simulink subsystem "AeroPropRefFranc"  (R2024b)
settings: Solver=VariableStepAuto  StartTime=0.0  StopTime=10.0  RelTol=1e-3
undefined symbols (not defined in the file or in its folder): ess, Force_b, Fprop_r, geom, H_b, Hdot_b, Moment_b, mot, mot2, mot3, mot4, Mprop_r, propel, propel2, propel3, propel4, pxf_diagram_options, SimIn, SimPar, tc, tc2, tc3, tc4
libraries: simulink x8, slpidlib x4, starslibAxisTransformations x2, libAxisTransformations x2
(part 2 of 10)

== system AeroPropRefFranc/Propulsion and Aerodynamic Forces and Moments/S-Function/Battery Model/powerplant/mot2 ==
  main_info_bus_in : Inport
  system_effort_in : Inport  Port=2
  system_flow_in : Inport  Port=3
  buscreator_system_bus_out1 : BusCreator  Inputs=2
  ctrl : Subsystem
  memoryctrl : Memory
  plant : Subsystem
      mask Display: disp('mot2_plant_map_Pelec_funTW_volt_in.slx')
  system_bus_out : Outport
  system_effort_out : Outport  Port=2
  system_flow_out : Outport  Port=3
  wires:
  [plant] -> buscreator_system_bus_out1/2  "plant"
  [ctrl] -> buscreator_system_bus_out1/1  "ctrl"
  buscreator_system_bus_out1/1 -> system_bus_out/1  "system_info_bus"
  system_flow_in/1 -> plant/4(in-flow-3)  "flow"
  system_effort_in/1 -> plant/3(in-effort-2)  "effort"
  plant/4(out-flow-8) -> system_flow_out/1  "flow"
  plant/3(out-effort-7) -> system_effort_out/1  "effort"
  plant/1(outport-system_info_bus) -> [plant]  "system_info_bus"
  memoryctrl/1 -> plant/2(inport-ctrl_bus-2)  "ctrl_bus"
  plant/2(outport-plant_bus) -> ctrl/2(local_info_bus_in)  "plant_bus"
  main_info_bus_in/1 -> plant/1(aInport--1), ctrl/1(main_info_bus_in)  "main_info_bus"
  ctrl/2(local_info_bus_out) -> memoryctrl/1  "ctrl_bus"
  ctrl/1(system_bus_out) -> [ctrl]  "system_info_bus"

== system AeroPropRefFranc/Propulsion and Aerodynamic Forces and Moments/S-Function/Battery Model/powerplant/mot3 ==
  main_info_bus_in : Inport
  system_effort_in : Inport  Port=2
  system_flow_in : Inport  Port=3
  buscreator_system_bus_out1 : BusCreator  Inputs=2
  ctrl : Subsystem
  memoryctrl : Memory
  plant : Subsystem
      mask Display: disp('mot3_plant_map_Pelec_funTW_volt_in.slx')
  system_bus_out : Outport
  system_effort_out : Outport  Port=2
  system_flow_out : Outport  Port=3
  wires:
  [plant] -> buscreator_system_bus_out1/2  "plant"
  [ctrl] -> buscreator_system_bus_out1/1  "ctrl"
  buscreator_system_bus_out1/1 -> system_bus_out/1  "system_info_bus"
  system_flow_in/1 -> plant/4(in-flow-3)  "flow"
  system_effort_in/1 -> plant/3(in-effort-2)  "effort"
  plant/4(out-flow-8) -> system_flow_out/1  "flow"
  plant/3(out-effort-7) -> system_effort_out/1  "effort"
  plant/1(outport-system_info_bus) -> [plant]  "system_info_bus"
  memoryctrl/1 -> plant/2(inport-ctrl_bus-2)  "ctrl_bus"
  plant/2(outport-plant_bus) -> ctrl/2(local_info_bus_in)  "plant_bus"
  main_info_bus_in/1 -> plant/1(aInport--1), ctrl/1(main_info_bus_in)  "main_info_bus"
  ctrl/2(local_info_bus_out) -> memoryctrl/1  "ctrl_bus"
  ctrl/1(system_bus_out) -> [ctrl]  "system_info_bus"

== system AeroPropRefFranc/Propulsion and Aerodynamic Forces and Moments/S-Function/Battery Model/powerplant/mot4 ==
  main_info_bus_in : Inport
  system_effort_in : Inport  Port=2
  system_flow_in : Inport  Port=3
  buscreator_system_bus_out1 : BusCreator  Inputs=2
  ctrl : Subsystem
  memoryctrl : Memory
  plant : Subsystem
      mask Display: disp('mot4_plant_map_Pelec_funTW_volt_in.slx')
  system_bus_out : Outport
  system_effort_out : Outport  Port=2
  system_flow_out : Outport  Port=3
  wires:
  [plant] -> buscreator_system_bus_out1/2  "plant"
  [ctrl] -> buscreator_system_bus_out1/1  "ctrl"
  buscreator_system_bus_out1/1 -> system_bus_out/1  "system_info_bus"
  system_flow_in/1 -> plant/4(in-flow-3)  "flow"
  system_effort_in/1 -> plant/3(in-effort-2)  "effort"
  plant/4(out-flow-8) -> system_flow_out/1  "flow"
  plant/3(out-effort-7) -> system_effort_out/1  "effort"
  plant/1(outport-system_info_bus) -> [plant]  "system_info_bus"
  memoryctrl/1 -> plant/2(inport-ctrl_bus-2)  "ctrl_bus"
  plant/2(outport-plant_bus) -> ctrl/2(local_info_bus_in)  "plant_bus"
  main_info_bus_in/1 -> plant/1(aInport--1), ctrl/1(main_info_bus_in)  "main_info_bus"
  ctrl/2(local_info_bus_out) -> memoryctrl/1  "ctrl_bus"
  ctrl/1(system_bus_out) -> [ctrl]  "system_info_bus"

== system AeroPropRefFranc/Propulsion and Aerodynamic Forces and Moments/S-Function/Battery Model/powerplant/propel ==
  main_info_bus_in : Inport
  system_effort_in : Inport  Port=2
  system_flow_in : Inport  Port=3
  Ground_1 : Ground
  Terminator_1 : Terminator
  plant : Subsystem
      mask Display: disp('propel_plant_uas.slx')
  system_bus_out : Outport
  system_effort_out : Outport  Port=2
  system_flow_out : Outport  Port=3
  wires:
  plant/2(aOutport--2) -> Terminator_1/1
  Ground_1/1 -> plant/2(aInport--2)
  [plant] -> system_bus_out/1  "plant"
  system_flow_in/1 -> plant/4(in-flow-5)
  system_effort_in/1 -> plant/3(in-effort-4)
  plant/4(out-flow-6) -> system_flow_out/1
  plant/3(out-effort-5) -> system_effort_out/1
  plant/1(outport-system_info_bus) -> [plant]
  main_info_bus_in/1 -> plant/1(inport-main_info_bus-1)

== system AeroPropRefFranc/Propulsion and Aerodynamic Forces and Moments/S-Function/Battery Model/powerplant/propel2 ==
  main_info_bus_in : Inport
  system_effort_in : Inport  Port=2
  system_flow_in : Inport  Port=3
  Ground_1 : Ground
  Terminator_1 : Terminator
  plant : Subsystem
      mask Display: disp('propel2_plant_uas.slx')
  system_bus_out : Outport
  system_effort_out : Outport  Port=2
  system_flow_out : Outport  Port=3
  wires:
  plant/2(aOutport--2) -> Terminator_1/1
  Ground_1/1 -> plant/2(aInport--2)
  [plant] -> system_bus_out/1  "plant"
  system_flow_in/1 -> plant/4(in-flow-5)
  system_effort_in/1 -> plant/3(in-effort-4)
  plant/4(out-flow-6) -> system_flow_out/1
  plant/3(out-effort-5) -> system_effort_out/1
  plant/1(outport-system_info_bus) -> [plant]
  main_info_bus_in/1 -> plant/1(inport-main_info_bus-1)

== system AeroPropRefFranc/Propulsion and Aerodynamic Forces and Moments/S-Function/Battery Model/powerplant/propel3 ==
  main_info_bus_in : Inport
  system_effort_in : Inport  Port=2
  system_flow_in : Inport  Port=3
  Ground_1 : Ground
  Terminator_1 : Terminator
  plant : Subsystem
      mask Display: disp('propel3_plant_uas.slx')
  system_bus_out : Outport
  system_effort_out : Outport  Port=2
  system_flow_out : Outport  Port=3
  wires:
  plant/2(aOutport--2) -> Terminator_1/1
  Ground_1/1 -> plant/2(aInport--2)
  [plant] -> system_bus_out/1  "plant"
  system_flow_in/1 -> plant/4(in-flow-5)
  system_effort_in/1 -> plant/3(in-effort-4)
  plant/4(out-flow-6) -> system_flow_out/1
  plant/3(out-effort-5) -> system_effort_out/1
  plant/1(outport-system_info_bus) -> [plant]
  main_info_bus_in/1 -> plant/1(inport-main_info_bus-1)

== system AeroPropRefFranc/Propulsion and Aerodynamic Forces and Moments/S-Function/Battery Model/powerplant/propel4 ==
  main_info_bus_in : Inport
  system_effort_in : Inport  Port=2
  system_flow_in : Inport  Port=3
  Ground_1 : Ground
  Terminator_1 : Terminator
  plant : Subsystem
      mask Display: disp('propel4_plant_uas.slx')
  system_bus_out : Outport
  system_effort_out : Outport  Port=2
  system_flow_out : Outport  Port=3
  wires:
  plant/2(aOutport--2) -> Terminator_1/1
  Ground_1/1 -> plant/2(aInport--2)
  [plant] -> system_bus_out/1  "plant"
  system_flow_in/1 -> plant/4(in-flow-5)
  system_effort_in/1 -> plant/3(in-effort-4)
  plant/4(out-flow-6) -> system_flow_out/1
  plant/3(out-effort-5) -> system_effort_out/1
  plant/1(outport-system_info_bus) -> [plant]
  main_info_bus_in/1 -> plant/1(inport-main_info_bus-1)

== system AeroPropRefFranc/Propulsion and Aerodynamic Forces and Moments/S-Function/Battery Model/powerplant/tc ==
  main_info_bus_in : Inport
  system_effort_in : Inport  Port=2
  system_flow_in : Inport  Port=3
  Ground_1 : Ground
  Terminator_1 : Terminator
  plant : Subsystem
      mask Display: disp('tc_plant_map_trqloss_funTW.slx')
  system_bus_out : Outport
  system_effort_out : Outport  Port=2
  system_flow_out : Outport  Port=3
  wires:
  plant/2(aOutport--2) -> Terminator_1/1
  Ground_1/1 -> plant/2(aInport--2)
  [plant] -> system_bus_out/1  "plant"
  system_flow_in/1 -> plant/4(in-flow-2)
  system_effort_in/1 -> plant/3(in-effort-1)
  plant/4(out-flow-8) -> system_flow_out/1
  plant/3(out-effort-7) -> system_effort_out/1
  plant/1(outport-system_info_bus) -> [plant]
  main_info_bus_in/1 -> plant/1(aInport--1)

== system AeroPropRefFranc/Propulsion and Aerodynamic Forces and Moments/S-Function/Battery Model/powerplant/tc2 ==
  main_info_bus_in : Inport
  system_effort_in : Inport  Port=2
  system_flow_in : Inport  Port=3
  Ground_1 : Ground
  Terminator_1 : Terminator
  plant : Subsystem
      mask Display: disp('tc2_plant_map_trqloss_funTW.slx')
  system_bus_out : Outport
  system_effort_out : Outport  Port=2
  system_flow_out : Outport  Port=3
  wires:
  plant/2(aOutport--2) -> Terminator_1/1
  Ground_1/1 -> plant/2(aInport--2)
  [plant] -> system_bus_out/1  "plant"
  system_flow_in/1 -> plant/4(in-flow-2)
  system_effort_in/1 -> plant/3(in-effort-1)
  plant/4(out-flow-8) -> system_flow_out/1
  plant/3(out-effort-7) -> system_effort_out/1
  plant/1(outport-system_info_bus) -> [plant]
  main_info_bus_in/1 -> plant/1(aInport--1)

== system AeroPropRefFranc/Propulsion and Aerodynamic Forces and Moments/S-Function/Battery Model/powerplant/tc3 ==
  main_info_bus_in : Inport
  system_effort_in : Inport  Port=2
  system_flow_in : Inport  Port=3
  Ground_1 : Ground
  Terminator_1 : Terminator
  plant : Subsystem
      mask Display: disp('tc3_plant_map_trqloss_funTW.slx')
  system_bus_out : Outport
  system_effort_out : Outport  Port=2
  system_flow_out : Outport  Port=3
  wires:
  plant/2(aOutport--2) -> Terminator_1/1
  Ground_1/1 -> plant/2(aInport--2)
  [plant] -> system_bus_out/1  "plant"
  system_flow_in/1 -> plant/4(in-flow-2)
  system_effort_in/1 -> plant/3(in-effort-1)
  plant/4(out-flow-8) -> system_flow_out/1
  plant/3(out-effort-7) -> system_effort_out/1
  plant/1(outport-system_info_bus) -> [plant]
  main_info_bus_in/1 -> plant/1(aInport--1)

== system AeroPropRefFranc/Propulsion and Aerodynamic Forces and Moments/S-Function/Battery Model/powerplant/tc4 ==
  main_info_bus_in : Inport
  system_effort_in : Inport  Port=2
  system_flow_in : Inport  Port=3
  Ground_1 : Ground
  Terminator_1 : Terminator
  plant : Subsystem
      mask Display: disp('tc4_plant_map_trqloss_funTW.slx')
  system_bus_out : Outport
  system_effort_out : Outport  Port=2
  system_flow_out : Outport  Port=3
  wires:
  plant/2(aOutport--2) -> Terminator_1/1
  Ground_1/1 -> plant/2(aInport--2)
  [plant] -> system_bus_out/1  "plant"
  system_flow_in/1 -> plant/4(in-flow-2)
  system_effort_in/1 -> plant/3(in-effort-1)
  plant/4(out-flow-8) -> system_flow_out/1
  plant/3(out-effort-7) -> system_effort_out/1
  plant/1(outport-system_info_bus) -> [plant]
  main_info_bus_in/1 -> plant/1(aInport--1)

== system AeroPropRefFranc/Propulsion and Aerodynamic Forces and Moments/S-Function/Battery Model/accelec/plant/accelec_plant_const_pwrloss_volt_in_nokey ==
  drv_key_on_dmd_simu : Inport
  accelec_volt_in : Inport  Port=2
  accelec_curr_out : Inport  Port=3
  Electrical Power : Constant  Value=accelec.plant.init.pwr
  Product : Product  Inputs=*/  InputSameDT=on  SaturateOnIntegerOverflow=on  OutDataTypeStr=Inherit: Same as first input
  Sum : Sum  InputSameDT=on  SaturateOnIntegerOverflow=on  OutDataTypeStr=Inherit: Same as first input
  Sum1 : Sum  InputSameDT=on  SaturateOnIntegerOverflow=on  OutDataTypeStr=Inherit: Same as first input
  Terminator : Terminator
  eps : Constant  Value=eps
  accelec_plant_volt_in_simu : Outport  VectorParamsAs1DForOutWhenUnconnected=off
  accelec_plant_pwr_simu : Outport  Port=2  VectorParamsAs1DForOutWhenUnconnected=off
  accelec_plant_curr_in_simu : Outport  Port=3  VectorParamsAs1DForOutWhenUnconnected=off
  accelec_plant_volt_out_simu : Outport  Port=4  VectorParamsAs1DForOutWhenUnconnected=off
  accelec_plant_curr_out_simu : Outport  Port=5  VectorParamsAs1DForOutWhenUnconnected=off
  accelec_volt_out : Outport  Port=6  VectorParamsAs1DForOutWhenUnconnected=off
  accelec_curr_in : Outport  Port=7  VectorParamsAs1DForOutWhenUnconnected=off
  wires:
  [accelec_plant_pwr_simu] -> accelec_plant_pwr_simu/1  "accelec_plant_pwr_simu"
  accelec_volt_in/1 -> Sum1/1, [accelec_plant_volt_in_simu], [accelec_plant_volt_out_simu], accelec_volt_out/1
  [accelec_plant_volt_in_simu] -> accelec_plant_volt_in_simu/1  "accelec_plant_volt_in_simu"
  eps/1 -> Sum1/2
  Product/1 -> [accelec_plant_curr_simu], Sum/1
  accelec_curr_out/1 -> [accelec_plant_curr_out_simu], Sum/2
  Sum/1 -> [accelec_plant_curr_in_simu], accelec_curr_in/1
  Sum1/1 -> Product/2
  [accelec_plant_curr_in_simu] -> accelec_plant_curr_in_simu/1  "accelec_plant_curr_in_simu"
  [accelec_plant_curr_out_simu] -> accelec_plant_curr_out_simu/1  "accelec_plant_curr_out_simu"
  [accelec_plant_volt_out_simu] -> accelec_plant_volt_out_simu/1  "accelec_plant_volt_out_simu"
  Electrical Power/1 -> [accelec_plant_pwr_simu], Product/1
  drv_key_on_dmd_simu/1 -> Terminator/1

== system AeroPropRefFranc/Propulsion and Aerodynamic Forces and Moments/S-Function/Battery Model/accelec/plant/parameter_out ==
  inport-accelec_plant_volt_in_simu : Inport
  inport-accelec_plant_pwr_simu : Inport  Port=2
  inport-accelec_plant_curr_in_simu : Inport  Port=3
  inport-accelec_plant_volt_out_simu : Inport  Port=4
  inport-accelec_plant_curr_out_simu : Inport  Port=5
  Ground_1 : Ground
  Toworkspace-accelec_plant_curr_in_simu : ToWorkspace  VariableName=accelec_plant_curr_in_simu  SampleTime=pxf_diagram_options.workspace_sample_time
      settings: Decimation=pxf_diagram_options.decimation
  Toworkspace-accelec_plant_curr_out_simu : ToWorkspace  VariableName=accelec_plant_curr_out_simu  SampleTime=pxf_diagram_options.workspace_sample_time
      settings: Decimation=pxf_diagram_options.decimation
  Toworkspace-accelec_plant_pwr_simu : ToWorkspace  VariableName=accelec_plant_pwr_simu  SampleTime=pxf_diagram_options.workspace_sample_time
      settings: Decimation=pxf_diagram_options.decimation
  Toworkspace-accelec_plant_volt_in_simu : ToWorkspace  VariableName=accelec_plant_volt_in_simu  SampleTime=pxf_diagram_options.workspace_sample_time
      settings: Decimation=pxf_diagram_options.decimation
  Toworkspace-accelec_plant_volt_out_simu : ToWorkspace  VariableName=accelec_plant_volt_out_simu  SampleTime=pxf_diagram_options.workspace_sample_time
      settings: Decimation=pxf_diagram_options.decimation
  outport-system_info_bus : Outport
  wires:
  Ground_1/1 -> outport-system_info_bus/1
  inport-accelec_plant_curr_out_simu/1 -> Toworkspace-accelec_plant_curr_out_simu/1
  inport-accelec_plant_volt_out_simu/1 -> Toworkspace-accelec_plant_volt_out_simu/1
  inport-accelec_plant_curr_in_simu/1 -> Toworkspace-accelec_plant_curr_in_simu/1
  inport-accelec_plant_pwr_simu/1 -> Toworkspace-accelec_plant_pwr_simu/1
  inport-accelec_plant_volt_in_simu/1 -> Toworkspace-accelec_plant_volt_in_simu/1

== system AeroPropRefFranc/Propulsion and Aerodynamic Forces and Moments/S-Function/Battery Model/accelec/plant/parameter_selection ==

== system AeroPropRefFranc/Propulsion and Aerodynamic Forces and Moments/S-Function/Battery Model/ess (battery)/ctrl/ess_ctrl_pngv_map_anl_PI_cstr ==
  ess_volt_out : Inport
  ess_curr_out : Inport  Port=2
  ess_soc : Inport  Port=3
  Demux : Demux  Outputs=3
  Demux1 : Demux  Outputs=3
  PI controller for maximal charge power and current1 : Subsystem
  PI controller for maximal discharge power and current1 : Subsystem
  mux1 : Mux  Inputs=3
  ess_ctrl_pwr_max_pro_simu : Outport
  ess_ctrl_pwr_max_reg_simu : Outport  Port=2
  ess_ctrl_curr_max_pro_simu : Outport  Port=3
  ess_ctrl_curr_max_reg_simu : Outport  Port=4
  wires:
  [ess_ctrl_pwr_max_reg_simu] -> ess_ctrl_pwr_max_reg_simu/1  "ess_ctrl_pwr_max_reg_simu"
  [ess_ctrl_pwr_max_pro_simu] -> ess_ctrl_pwr_max_pro_simu/1  "ess_ctrl_pwr_max_pro_simu"
  [ess_ctrl_curr_max_pro_simu] -> ess_ctrl_curr_max_pro_simu/1  "ess_ctrl_curr_max_pro_simu"
  [ess_ctrl_curr_max_reg_simu] -> ess_ctrl_curr_max_reg_simu/1  "ess_ctrl_curr_max_reg_simu"
  PI controller for maximal discharge power and current1/1(Curr_max_prop) -> [ess_ctrl_curr_max_pro_simu]
  PI controller for maximal charge power and current1/2(Curr_max_reg) -> [ess_ctrl_curr_max_reg_simu]
  ess_volt_out/1 -> mux1/1  "ess_plant_volt_out_simu"
  mux1/1 -> Demux/1, Demux1/1
  PI controller for maximal discharge power and current1/2(Pwr_max_prop) -> [ess_ctrl_pwr_max_pro_simu]
  PI controller for maximal charge power and current1/1(Pwr_max_reg) -> [ess_ctrl_pwr_max_reg_simu]
  Demux/1 -> PI controller for maximal discharge power and current1/1(ess voltage)
  Demux/2 -> PI controller for maximal discharge power and current1/2(ess curr)
  Demux/3 -> PI controller for maximal discharge power and current1/3(SOC)
  Demux1/1 -> PI controller for maximal charge power and current1/1(ess voltage)
  Demux1/2 -> PI controller for maximal charge power and current1/2(ess curr)
  Demux1/3 -> PI controller for maximal charge power and current1/3(SOC)
  ess_curr_out/1 -> mux1/2  "ess_plant_curr_out_simu"
  ess_soc/1 -> mux1/3  "ess_plant_soc_simu"

== system AeroPropRefFranc/Propulsion and Aerodynamic Forces and Moments/S-Function/Battery Model/ess (battery)/ctrl/parameter_out ==
  inport-ess_ctrl_pwr_max_pro_simu : Inport
  inport-ess_ctrl_pwr_max_reg_simu : Inport  Port=2
  inport-ess_ctrl_curr_max_pro_simu : Inport  Port=3
  inport-ess_ctrl_curr_max_reg_simu : Inport  Port=4
  Ground_1 : Ground
  Toworkspace-ess_ctrl_curr_max_pro_simu : ToWorkspace  Commented=on  VariableName=ess_ctrl_curr_max_pro_simu  SampleTime=pxf_diagram_options.workspace_sample_time
      settings: Decimation=pxf_diagram_options.decimation
  Toworkspace-ess_ctrl_curr_max_reg_simu : ToWorkspace  Commented=on  VariableName=ess_ctrl_curr_max_reg_simu  SampleTime=pxf_diagram_options.workspace_sample_time
      settings: Decimation=pxf_diagram_options.decimation
  Toworkspace-ess_ctrl_pwr_max_pro_simu : ToWorkspace  Commented=on  VariableName=ess_ctrl_pwr_max_pro_simu  SampleTime=pxf_diagram_options.workspace_sample_time
      settings: Decimation=pxf_diagram_options.decimation
  Toworkspace-ess_ctrl_pwr_max_reg_simu : ToWorkspace  Commented=on  VariableName=ess_ctrl_pwr_max_reg_simu  SampleTime=pxf_diagram_options.workspace_sample_time
      settings: Decimation=pxf_diagram_options.decimation
  create_system_info_bus : BusCreator  Inputs=1
  outport-system_info_bus : Outport
  outport-ctrl_bus : Outport  Port=2
  wires:
  Ground_1/1 -> outport-ctrl_bus/1
  inport-ess_ctrl_curr_max_reg_simu/1 -> Toworkspace-ess_ctrl_curr_max_reg_simu/1
  inport-ess_ctrl_curr_max_pro_simu/1 -> Toworkspace-ess_ctrl_curr_max_pro_simu/1
  inport-ess_ctrl_pwr_max_reg_simu/1 -> Toworkspace-ess_ctrl_pwr_max_reg_simu/1
  inport-ess_ctrl_pwr_max_pro_simu/1 -> Toworkspace-ess_ctrl_pwr_max_pro_simu/1, create_system_info_bus/1  "ess_ctrl_pwr_max_pro_simu"
  create_system_info_bus/1 -> outport-system_info_bus/1

== system AeroPropRefFranc/Propulsion and Aerodynamic Forces and Moments/S-Function/Battery Model/ess (battery)/ctrl/parameter_selection ==
  inport-main_info_bus-1 : Inport
  select_main_info_bus : BusSelector  OutputSignals=plant.ess_plant_volt_out_simu,plant.ess_plant_curr_out_simu,plant.ess_plant_soc_simu
  outport-ess_plant_volt_out_simu-1 : Outport
  outport-ess_plant_curr_out_simu-2 : Outport  Port=2
  outport-ess_plant_soc_simu-3 : Outport  Port=3
  wires:
  select_main_info_bus/3 -> outport-ess_plant_soc_simu-3/1  "<ess_plant_soc_simu>"
  select_main_info_bus/2 -> outport-ess_plant_curr_out_simu-2/1  "<ess_plant_curr_out_simu>"
  select_main_info_bus/1 -> outport-ess_plant_volt_out_simu-1/1  "<ess_plant_volt_out_simu>"
  inport-main_info_bus-1/1 -> select_main_info_bus/1

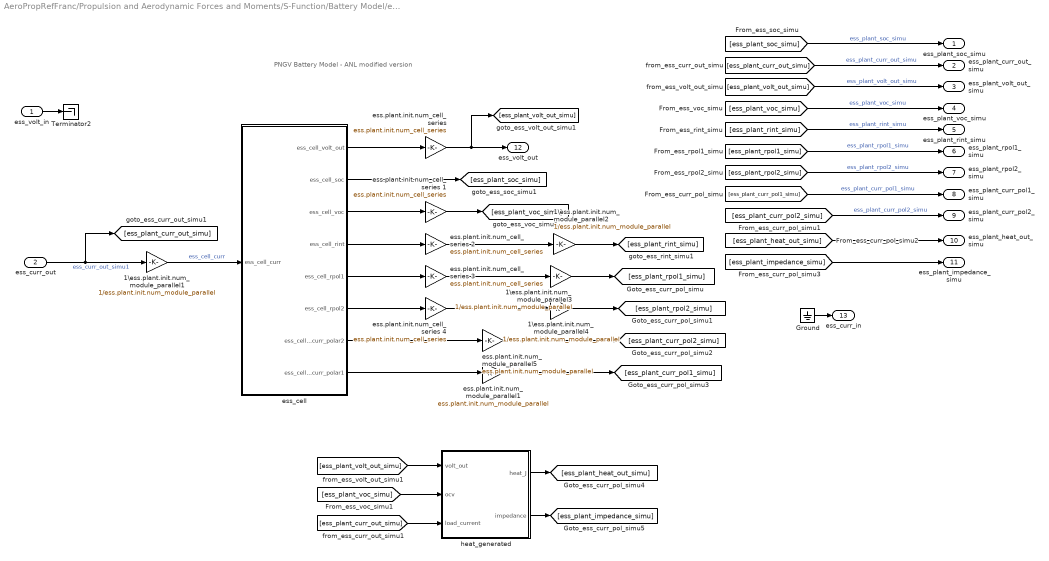
== system AeroPropRefFranc/Propulsion and Aerodynamic Forces and Moments/S-Function/Battery Model/ess (battery)/plant/ess_plant_pngv_map_anl_PI_cstr ==
  note: PNGV Battery Model - ANL modified version
  ess_volt_in : Inport
  ess_curr_out : Inport  Port=2
  1\ess.plant.init.num_module_parallel{1..4} (4 alike) : Gain  Gain=1/ess.plant.init.num_module_parallel
  Ground : Ground
  Terminator2 : Terminator
  ess.plant.init.num_cell_series {,1..4} (5 alike) : Gain  Gain=ess.plant.init.num_cell_series
  ess.plant.init.num_module_parallel1 : Gain  Gain=ess.plant.init.num_module_parallel
  ess.plant.init.num_module_parallel5 : Gain  Gain=ess.plant.init.num_module_parallel
  ess_cell : Subsystem
  heat_generated : Subsystem
  ess_plant_soc_simu : Outport
  ess_plant_curr_out_simu : Outport  Port=2
  ess_plant_volt_out_simu : Outport  Port=3
  ess_plant_voc_simu : Outport  Port=4
  ess_plant_rint_simu : Outport  Port=5
  ess_plant_rpol1_simu : Outport  Port=6
  ess_plant_rpol2_simu : Outport  Port=7
  ess_plant_curr_pol1_simu : Outport  Port=8
  ess_plant_curr_pol2_simu : Outport  Port=9
  ess_plant_heat_out_simu : Outport  Port=10
  ess_plant_impedance_simu : Outport  Port=11
  ess_volt_out : Outport  Port=12
  ess_curr_in : Outport  Port=13
  wires:
  Ground/1 -> ess_curr_in/1
  ess_volt_in/1 -> Terminator2/1
  [ess_plant_soc_simu] -> ess_plant_soc_simu/1  "ess_plant_soc_simu"
  [ess_plant_curr_out_simu] -> ess_plant_curr_out_simu/1  "ess_plant_curr_out_simu"
  [ess_plant_volt_out_simu] -> ess_plant_volt_out_simu/1  "ess_plant_volt_out_simu"
  [ess_plant_voc_simu] -> ess_plant_voc_simu/1  "ess_plant_voc_simu"
  [ess_plant_rint_simu] -> ess_plant_rint_simu/1  "ess_plant_rint_simu"
  [ess_plant_rpol1_simu] -> ess_plant_rpol1_simu/1  "ess_plant_rpol1_simu"
  [ess_plant_rpol2_simu] -> ess_plant_rpol2_simu/1  "ess_plant_rpol2_simu"
  [ess_plant_curr_pol1_simu] -> ess_plant_curr_pol1_simu/1  "ess_plant_curr_pol1_simu"
  [ess_plant_curr_pol2_simu] -> ess_plant_curr_pol2_simu/1  "ess_plant_curr_pol2_simu"
  ess_cell/1(ess_cell_volt_out) -> "ess.plant.init.num_cell_series "/1
  1\ess.plant.init.num_module_parallel1/1 -> ess_cell/1(ess_cell_curr)  "ess_cell_curr"
  "ess.plant.init.num_cell_series "/1 -> [ess_plant_volt_out_simu], ess_volt_out/1
  ess.plant.init.num_cell_series 2/1 -> 1\ess.plant.init.num_module_parallel2/1
  ess.plant.init.num_cell_series 1/1 -> [ess_plant_voc_simu]
  1\ess.plant.init.num_module_parallel2/1 -> [ess_plant_rint_simu]
  ess_curr_out/1 -> 1\ess.plant.init.num_module_parallel1/1, [ess_plant_curr_out_simu]  "ess_curr_out_simu1"
  ess_cell/3(ess_cell_voc) -> ess.plant.init.num_cell_series 1/1
  ess_cell/4(ess_cell_rint) -> ess.plant.init.num_cell_series 2/1
  ess_cell/2(ess_cell_soc) -> [ess_plant_soc_simu]
  ess_cell/5(ess_cell_rpol1) -> ess.plant.init.num_cell_series 3/1
  ess_cell/6(ess_cell_rpol2) -> ess.plant.init.num_cell_series 4/1
  ess.plant.init.num_cell_series 3/1 -> 1\ess.plant.init.num_module_parallel3/1
  1\ess.plant.init.num_module_parallel3/1 -> [ess_plant_rpol1_simu]
  ess.plant.init.num_cell_series 4/1 -> 1\ess.plant.init.num_module_parallel4/1
  1\ess.plant.init.num_module_parallel4/1 -> [ess_plant_rpol2_simu]
  ess_cell/8(ess_cell_curr_polar1) -> ess.plant.init.num_module_parallel1/1
  ess_cell/7(ess_cell_curr_polar2) -> ess.plant.init.num_module_parallel5/1
  ess.plant.init.num_module_parallel5/1 -> [ess_plant_curr_pol2_simu]
  ess.plant.init.num_module_parallel1/1 -> [ess_plant_curr_pol1_simu]
  [ess_plant_volt_out_simu] -> heat_generated/1(volt_out)
  [ess_plant_voc_simu] -> heat_generated/2(ocv)
  [ess_plant_curr_out_simu] -> heat_generated/3(load_current)
  heat_generated/1(heat_J) -> [ess_plant_heat_out_simu]
  [ess_plant_heat_out_simu] -> ess_plant_heat_out_simu/1
  heat_generated/2(impedance) -> [ess_plant_impedance_simu]
  [ess_plant_impedance_simu] -> ess_plant_impedance_simu/1

== system AeroPropRefFranc/Propulsion and Aerodynamic Forces and Moments/S-Function/Battery Model/ess (battery)/plant/parameter_out ==
  inport-ess_plant_soc_simu : Inport
  inport-ess_plant_curr_out_simu : Inport  Port=2
  inport-ess_plant_volt_out_simu : Inport  Port=3
  inport-ess_plant_voc_simu : Inport  Port=4
  inport-ess_plant_rint_simu : Inport  Port=5
  inport-ess_plant_rpol1_simu : Inport  Port=6
  inport-ess_plant_rpol2_simu : Inport  Port=7
  inport-ess_plant_curr_pol1_simu : Inport  Port=8
  inport-ess_plant_curr_pol2_simu : Inport  Port=9
  inport-ess_plant_heat_out_simu : Inport  Port=10
  inport-ess_plant_impedance_simu : Inport  Port=11
  Ground_1 : Ground
  Toworkspace-ess_plant_curr_out_simu : ToWorkspace  VariableName=ess_plant_curr_out_simu  SampleTime=pxf_diagram_options.workspace_sample_time
      settings: Decimation=pxf_diagram_options.decimation
  Toworkspace-ess_plant_curr_pol1_simu : ToWorkspace  VariableName=ess_plant_curr_pol1_simu  SampleTime=pxf_diagram_options.workspace_sample_time
      settings: Decimation=pxf_diagram_options.decimation
  Toworkspace-ess_plant_curr_pol2_simu : ToWorkspace  VariableName=ess_plant_curr_pol2_simu  SampleTime=pxf_diagram_options.workspace_sample_time
      settings: Decimation=pxf_diagram_options.decimation
  Toworkspace-ess_plant_heat_out_simu : ToWorkspace  VariableName=ess_plant_heat_out_simu  SampleTime=pxf_diagram_options.workspace_sample_time
      settings: Decimation=pxf_diagram_options.decimation
  Toworkspace-ess_plant_impedance_simu : ToWorkspace  VariableName=ess_plant_impedance_simu  SampleTime=pxf_diagram_options.workspace_sample_time
      settings: Decimation=pxf_diagram_options.decimation
  Toworkspace-ess_plant_rint_simu : ToWorkspace  VariableName=ess_plant_rint_simu  SampleTime=pxf_diagram_options.workspace_sample_time
      settings: Decimation=pxf_diagram_options.decimation
  Toworkspace-ess_plant_rpol1_simu : ToWorkspace  VariableName=ess_plant_rpol1_simu  SampleTime=pxf_diagram_options.workspace_sample_time
      settings: Decimation=pxf_diagram_options.decimation
  Toworkspace-ess_plant_rpol2_simu : ToWorkspace  VariableName=ess_plant_rpol2_simu  SampleTime=pxf_diagram_options.workspace_sample_time
      settings: Decimation=pxf_diagram_options.decimation
  Toworkspace-ess_plant_soc_simu : ToWorkspace  VariableName=ess_plant_soc_simu  SampleTime=pxf_diagram_options.workspace_sample_time
      settings: Decimation=pxf_diagram_options.decimation
  Toworkspace-ess_plant_voc_simu : ToWorkspace  VariableName=ess_plant_voc_simu  SampleTime=pxf_diagram_options.workspace_sample_time
      settings: Decimation=pxf_diagram_options.decimation
  Toworkspace-ess_plant_volt_out_simu : ToWorkspace  VariableName=ess_plant_volt_out_simu  SampleTime=pxf_diagram_options.workspace_sample_time
      settings: Decimation=pxf_diagram_options.decimation
  create_system_info_bus : BusCreator  Inputs=3
  outport-system_info_bus : Outport
  outport-plant_bus : Outport  Port=2
  wires:
  Ground_1/1 -> outport-plant_bus/1
  inport-ess_plant_curr_pol2_simu/1 -> Toworkspace-ess_plant_curr_pol2_simu/1
  inport-ess_plant_curr_pol1_simu/1 -> Toworkspace-ess_plant_curr_pol1_simu/1
  inport-ess_plant_rpol2_simu/1 -> Toworkspace-ess_plant_rpol2_simu/1
  inport-ess_plant_rpol1_simu/1 -> Toworkspace-ess_plant_rpol1_simu/1
  inport-ess_plant_rint_simu/1 -> Toworkspace-ess_plant_rint_simu/1
  inport-ess_plant_voc_simu/1 -> Toworkspace-ess_plant_voc_simu/1
  inport-ess_plant_volt_out_simu/1 -> Toworkspace-ess_plant_volt_out_simu/1, create_system_info_bus/3  "ess_plant_volt_out_simu"
  inport-ess_plant_curr_out_simu/1 -> Toworkspace-ess_plant_curr_out_simu/1, create_system_info_bus/2  "ess_plant_curr_out_simu"
  inport-ess_plant_impedance_simu/1 -> Toworkspace-ess_plant_impedance_simu/1
  inport-ess_plant_heat_out_simu/1 -> Toworkspace-ess_plant_heat_out_simu/1
  inport-ess_plant_soc_simu/1 -> Toworkspace-ess_plant_soc_simu/1, create_system_info_bus/1  "ess_plant_soc_simu"
  create_system_info_bus/1 -> outport-system_info_bus/1

== system AeroPropRefFranc/Propulsion and Aerodynamic Forces and Moments/S-Function/Battery Model/ess (battery)/plant/parameter_selection ==

== system AeroPropRefFranc/Propulsion and Aerodynamic Forces and Moments/S-Function/Battery Model/powerplant/accelec/plant ==
  aInport--1 : Inport
  aInport--2 : Inport  Port=2
  in-effort-2 : Inport  Port=3
  in-flow-3 : Inport  Port=4
  Ground_1 : Ground
  Ground_2 : Ground
  Terminator_1 : Terminator
  Terminator_2 : Terminator
  accelec_plant_const_pwrloss_volt_in_nokey : Subsystem
  parameter_out : Subsystem
  parameter_selection : Subsystem
  outport-system_info_bus : Outport
  aOutport--2 : Outport  Port=2
  out-effort-6 : Outport  Port=3
  out-flow-7 : Outport  Port=4
  wires:
  Ground_2/1 -> aOutport--2/1
  Ground_1/1 -> accelec_plant_const_pwrloss_volt_in_nokey/1(drv_key_on_dmd_simu)
  aInport--2/1 -> Terminator_2/1
  aInport--1/1 -> Terminator_1/1
  accelec_plant_const_pwrloss_volt_in_nokey/7(accelec_curr_in) -> out-flow-7/1
  accelec_plant_const_pwrloss_volt_in_nokey/6(accelec_volt_out) -> out-effort-6/1
  in-flow-3/1 -> accelec_plant_const_pwrloss_volt_in_nokey/3(accelec_curr_out)
  in-effort-2/1 -> accelec_plant_const_pwrloss_volt_in_nokey/2(accelec_volt_in)
  accelec_plant_const_pwrloss_volt_in_nokey/5(accelec_plant_curr_out_simu) -> parameter_out/5(inport-accelec_plant_curr_out_simu)
  accelec_plant_const_pwrloss_volt_in_nokey/4(accelec_plant_volt_out_simu) -> parameter_out/4(inport-accelec_plant_volt_out_simu)
  accelec_plant_const_pwrloss_volt_in_nokey/3(accelec_plant_curr_in_simu) -> parameter_out/3(inport-accelec_plant_curr_in_simu)
  accelec_plant_const_pwrloss_volt_in_nokey/2(accelec_plant_pwr_simu) -> parameter_out/2(inport-accelec_plant_pwr_simu)
  accelec_plant_const_pwrloss_volt_in_nokey/1(accelec_plant_volt_in_simu) -> parameter_out/1(inport-accelec_plant_volt_in_simu)
  parameter_out/1(outport-system_info_bus) -> outport-system_info_bus/1

== system AeroPropRefFranc/Propulsion and Aerodynamic Forces and Moments/S-Function/Battery Model/powerplant/ess (battery)/ctrl ==
  inport-main_info_bus-1 : Inport
  aInport--2 : Inport  Port=2
  Terminator_1 : Terminator
  ess_ctrl_pngv_map_anl_PI_cstr : Subsystem
  parameter_out : Subsystem
  parameter_selection : Subsystem
  outport-system_info_bus : Outport
  outport-ctrl_bus : Outport  Port=2
  wires:
  aInport--2/1 -> Terminator_1/1
  parameter_selection/3(outport-ess_plant_soc_simu-3) -> ess_ctrl_pngv_map_anl_PI_cstr/3(ess_soc)
  parameter_selection/2(outport-ess_plant_curr_out_simu-2) -> ess_ctrl_pngv_map_anl_PI_cstr/2(ess_curr_out)
  parameter_selection/1(outport-ess_plant_volt_out_simu-1) -> ess_ctrl_pngv_map_anl_PI_cstr/1(ess_volt_out)
  ess_ctrl_pngv_map_anl_PI_cstr/4(ess_ctrl_curr_max_reg_simu) -> parameter_out/4(inport-ess_ctrl_curr_max_reg_simu)
  ess_ctrl_pngv_map_anl_PI_cstr/3(ess_ctrl_curr_max_pro_simu) -> parameter_out/3(inport-ess_ctrl_curr_max_pro_simu)
  ess_ctrl_pngv_map_anl_PI_cstr/2(ess_ctrl_pwr_max_reg_simu) -> parameter_out/2(inport-ess_ctrl_pwr_max_reg_simu)
  ess_ctrl_pngv_map_anl_PI_cstr/1(ess_ctrl_pwr_max_pro_simu) -> parameter_out/1(inport-ess_ctrl_pwr_max_pro_simu)
  parameter_out/2(outport-ctrl_bus) -> outport-ctrl_bus/1
  parameter_out/1(outport-system_info_bus) -> outport-system_info_bus/1
  inport-main_info_bus-1/1 -> parameter_selection/1(inport-main_info_bus-1)

== system AeroPropRefFranc/Propulsion and Aerodynamic Forces and Moments/S-Function/Battery Model/powerplant/ess (battery)/plant ==
  aInport--1 : Inport
  aInport--2 : Inport  Port=2
  in-effort-1 : Inport  Port=3
  in-flow-2 : Inport  Port=4
  Terminator_1 : Terminator
  Terminator_2 : Terminator
  ess_plant_pngv_map_anl_PI_cstr : Subsystem
  parameter_out : Subsystem
  parameter_selection : Subsystem
  outport-system_info_bus : Outport
  outport-plant_bus : Outport  Port=2
  out-effort-12 : Outport  Port=3
  out-flow-13 : Outport  Port=4
  wires:
  aInport--2/1 -> Terminator_2/1
  aInport--1/1 -> Terminator_1/1
  ess_plant_pngv_map_anl_PI_cstr/13(ess_curr_in) -> out-flow-13/1
  ess_plant_pngv_map_anl_PI_cstr/12(ess_volt_out) -> out-effort-12/1
  in-flow-2/1 -> ess_plant_pngv_map_anl_PI_cstr/2(ess_curr_out)
  in-effort-1/1 -> ess_plant_pngv_map_anl_PI_cstr/1(ess_volt_in)
  ess_plant_pngv_map_anl_PI_cstr/9(ess_plant_curr_pol2_simu) -> parameter_out/9(inport-ess_plant_curr_pol2_simu)
  ess_plant_pngv_map_anl_PI_cstr/8(ess_plant_curr_pol1_simu) -> parameter_out/8(inport-ess_plant_curr_pol1_simu)
  ess_plant_pngv_map_anl_PI_cstr/7(ess_plant_rpol2_simu) -> parameter_out/7(inport-ess_plant_rpol2_simu)
  ess_plant_pngv_map_anl_PI_cstr/6(ess_plant_rpol1_simu) -> parameter_out/6(inport-ess_plant_rpol1_simu)
  ess_plant_pngv_map_anl_PI_cstr/5(ess_plant_rint_simu) -> parameter_out/5(inport-ess_plant_rint_simu)
  ess_plant_pngv_map_anl_PI_cstr/4(ess_plant_voc_simu) -> parameter_out/4(inport-ess_plant_voc_simu)
  ess_plant_pngv_map_anl_PI_cstr/3(ess_plant_volt_out_simu) -> parameter_out/3(inport-ess_plant_volt_out_simu)
  ess_plant_pngv_map_anl_PI_cstr/2(ess_plant_curr_out_simu) -> parameter_out/2(inport-ess_plant_curr_out_simu)
  ess_plant_pngv_map_anl_PI_cstr/11(ess_plant_impedance_simu) -> parameter_out/11(inport-ess_plant_impedance_simu)
  ess_plant_pngv_map_anl_PI_cstr/10(ess_plant_heat_out_simu) -> parameter_out/10(inport-ess_plant_heat_out_simu)
  ess_plant_pngv_map_anl_PI_cstr/1(ess_plant_soc_simu) -> parameter_out/1(inport-ess_plant_soc_simu)
  parameter_out/2(outport-plant_bus) -> outport-plant_bus/1
  parameter_out/1(outport-system_info_bus) -> outport-system_info_bus/1

== system AeroPropRefFranc/Propulsion and Aerodynamic Forces and Moments/S-Function/Battery Model/powerplant/ess (battery)1/ctrl ==
  inport-main_info_bus-1 : Inport
  aInport--2 : Inport  Port=2
  Terminator_1 : Terminator
  ess_ctrl_pngv_map_anl_PI_cstr : Subsystem
  parameter_out : Subsystem
  parameter_selection : Subsystem
  outport-system_info_bus : Outport
  outport-ctrl_bus : Outport  Port=2
  wires:
  inport-main_info_bus-1/1 -> parameter_selection/1(inport-main_info_bus-1)
  parameter_out/1(outport-system_info_bus) -> outport-system_info_bus/1
  parameter_out/2(outport-ctrl_bus) -> outport-ctrl_bus/1
  ess_ctrl_pngv_map_anl_PI_cstr/1(ess_ctrl_pwr_max_pro_simu) -> parameter_out/1(inport-ess_ctrl_pwr_max_pro_simu)
  ess_ctrl_pngv_map_anl_PI_cstr/2(ess_ctrl_pwr_max_reg_simu) -> parameter_out/2(inport-ess_ctrl_pwr_max_reg_simu)
  ess_ctrl_pngv_map_anl_PI_cstr/3(ess_ctrl_curr_max_pro_simu) -> parameter_out/3(inport-ess_ctrl_curr_max_pro_simu)
  ess_ctrl_pngv_map_anl_PI_cstr/4(ess_ctrl_curr_max_reg_simu) -> parameter_out/4(inport-ess_ctrl_curr_max_reg_simu)
  parameter_selection/1(outport-ess_plant_volt_out_simu-1) -> ess_ctrl_pngv_map_anl_PI_cstr/1(ess_volt_out)
  parameter_selection/2(outport-ess_plant_curr_out_simu-2) -> ess_ctrl_pngv_map_anl_PI_cstr/2(ess_curr_out)
  parameter_selection/3(outport-ess_plant_soc_simu-3) -> ess_ctrl_pngv_map_anl_PI_cstr/3(ess_soc)
  aInport--2/1 -> Terminator_1/1

== system AeroPropRefFranc/Propulsion and Aerodynamic Forces and Moments/S-Function/Battery Model/powerplant/ess (battery)1/plant ==
  aInport--1 : Inport
  aInport--2 : Inport  Port=2
  in-effort-1 : Inport  Port=3
  in-flow-2 : Inport  Port=4
  Terminator_1 : Terminator
  Terminator_2 : Terminator
  ess_plant_pngv_map_anl_PI_cstr : Subsystem
  parameter_out : Subsystem
  parameter_selection : Subsystem
  outport-system_info_bus : Outport
  outport-plant_bus : Outport  Port=2
  out-effort-12 : Outport  Port=3
  out-flow-13 : Outport  Port=4
  wires:
  parameter_out/1(outport-system_info_bus) -> outport-system_info_bus/1
  parameter_out/2(outport-plant_bus) -> outport-plant_bus/1
  ess_plant_pngv_map_anl_PI_cstr/1(ess_plant_soc_simu) -> parameter_out/1(inport-ess_plant_soc_simu)
  ess_plant_pngv_map_anl_PI_cstr/10(ess_plant_heat_out_simu) -> parameter_out/10(inport-ess_plant_heat_out_simu)
  ess_plant_pngv_map_anl_PI_cstr/11(ess_plant_impedance_simu) -> parameter_out/11(inport-ess_plant_impedance_simu)
  ess_plant_pngv_map_anl_PI_cstr/2(ess_plant_curr_out_simu) -> parameter_out/2(inport-ess_plant_curr_out_simu)
  ess_plant_pngv_map_anl_PI_cstr/3(ess_plant_volt_out_simu) -> parameter_out/3(inport-ess_plant_volt_out_simu)
  ess_plant_pngv_map_anl_PI_cstr/4(ess_plant_voc_simu) -> parameter_out/4(inport-ess_plant_voc_simu)
  ess_plant_pngv_map_anl_PI_cstr/5(ess_plant_rint_simu) -> parameter_out/5(inport-ess_plant_rint_simu)
  ess_plant_pngv_map_anl_PI_cstr/6(ess_plant_rpol1_simu) -> parameter_out/6(inport-ess_plant_rpol1_simu)
  ess_plant_pngv_map_anl_PI_cstr/7(ess_plant_rpol2_simu) -> parameter_out/7(inport-ess_plant_rpol2_simu)
  ess_plant_pngv_map_anl_PI_cstr/8(ess_plant_curr_pol1_simu) -> parameter_out/8(inport-ess_plant_curr_pol1_simu)
  ess_plant_pngv_map_anl_PI_cstr/9(ess_plant_curr_pol2_simu) -> parameter_out/9(inport-ess_plant_curr_pol2_simu)
  in-effort-1/1 -> ess_plant_pngv_map_anl_PI_cstr/1(ess_volt_in)
  in-flow-2/1 -> ess_plant_pngv_map_anl_PI_cstr/2(ess_curr_out)
  ess_plant_pngv_map_anl_PI_cstr/12(ess_volt_out) -> out-effort-12/1
  ess_plant_pngv_map_anl_PI_cstr/13(ess_curr_in) -> out-flow-13/1
  aInport--1/1 -> Terminator_1/1
  aInport--2/1 -> Terminator_2/1

== system AeroPropRefFranc/Propulsion and Aerodynamic Forces and Moments/S-Function/Battery Model/powerplant/mot/ctrl ==
  main_info_bus_in : Inport
  local_info_bus_in : Inport  Port=2
  buscreator_system_bus_out1 : BusCreator  Inputs=3
  cmd : Subsystem
      mask Display: disp('mot_ctrl_cmd_map_Pelec_funTW_volt_in.slx')
  cstr : Subsystem
      mask Display: disp('mot_ctrl_cstr_map_Pelec_funTW_volt_in.slx')
  dmd : Subsystem
      mask Display: disp('mot_ctrl_dmd_uas.slx')
  system_bus_out : Outport
  local_info_bus_out : Outport  Port=2
  wires:
  [dmd] -> buscreator_system_bus_out1/3  "dmd"
  [cstr] -> buscreator_system_bus_out1/2  "cstr"
  [cmd] -> buscreator_system_bus_out1/1  "cmd"
  buscreator_system_bus_out1/1 -> system_bus_out/1
  local_info_bus_in/1 -> [local_info_bus]
  main_info_bus_in/1 -> [main_info_bus]
  [main_info_bus] -> cmd/1(inport-main_info_bus-1)
  [local_info_bus] -> cmd/2(aInport--2)
  cmd/1(outport-system_info_bus) -> [cmd], local_info_bus_out/1
  [main_info_bus] -> cstr/1(inport-main_info_bus-1)
  [local_info_bus] -> cstr/2(aInport--2)
  cstr/2(outport-cstr_bus) -> cmd/3(aInport--3)
  cstr/1(outport-system_info_bus) -> [cstr]
  [main_info_bus] -> dmd/1(inport-main_info_bus-1)
  [local_info_bus] -> dmd/2(aInport--2)
  dmd/2(outport-dmd_bus) -> cstr/3(aInport--3), cmd/4(aInport--4)
  dmd/1(outport-system_info_bus) -> [dmd]

== system AeroPropRefFranc/Propulsion and Aerodynamic Forces and Moments/S-Function/Battery Model/powerplant/mot/plant ==
  aInport--1 : Inport
  inport-ctrl_bus-2 : Inport  Port=2
  in-effort-2 : Inport  Port=3
  in-flow-3 : Inport  Port=4
  Ground_1 : Ground
  Terminator_1 : Terminator
  mot_plant_map_Pelec_funTW_volt_in : Subsystem
  parameter_out : Subsystem
  parameter_selection : Subsystem
  outport-system_info_bus : Outport
  outport-plant_bus : Outport  Port=2
  out-effort-7 : Outport  Port=3
  out-flow-8 : Outport  Port=4
  wires:
  Ground_1/1 -> parameter_selection/1(Inport_1)
  aInport--1/1 -> Terminator_1/1
  mot_plant_map_Pelec_funTW_volt_in/8(mot_current_out) -> out-flow-8/1
  mot_plant_map_Pelec_funTW_volt_in/7(mot_trq_out mot_inertia_out) -> out-effort-7/1
  in-flow-3/1 -> mot_plant_map_Pelec_funTW_volt_in/3(spd)
  in-effort-2/1 -> mot_plant_map_Pelec_funTW_volt_in/2(voltage)
  parameter_selection/1(outport-mot_ctrl_cmd_simu-1) -> mot_plant_map_Pelec_funTW_volt_in/1(mot_ctrl_cmd_simu)
  mot_plant_map_Pelec_funTW_volt_in/6(mot_plant_temp_coeff_simu) -> parameter_out/6(inport-mot_plant_temp_coeff_simu)
  mot_plant_map_Pelec_funTW_volt_in/5(mot_plant_trq_out_simu) -> parameter_out/5(inport-mot_plant_trq_out_simu)
  mot_plant_map_Pelec_funTW_volt_in/4(mot_plant_cmd_simu) -> parameter_out/4(inport-mot_plant_cmd_simu)
  mot_plant_map_Pelec_funTW_volt_in/3(mot_plant_volt_in_simu) -> parameter_out/3(inport-mot_plant_volt_in_simu)
  mot_plant_map_Pelec_funTW_volt_in/2(mot_plant_curr_in_simu) -> parameter_out/2(inport-mot_plant_curr_in_simu)
  mot_plant_map_Pelec_funTW_volt_in/1(mot_plant_spd_out_simu) -> parameter_out/1(inport-mot_plant_spd_out_simu)
  parameter_out/2(outport-plant_bus) -> outport-plant_bus/1
  parameter_out/1(outport-system_info_bus) -> outport-system_info_bus/1
  inport-ctrl_bus-2/1 -> parameter_selection/2(inport-ctrl_bus-2)

== system AeroPropRefFranc/Propulsion and Aerodynamic Forces and Moments/S-Function/Battery Model/powerplant/mot2/ctrl ==
  main_info_bus_in : Inport
  local_info_bus_in : Inport  Port=2
  buscreator_system_bus_out1 : BusCreator  Inputs=3
  cmd : Subsystem
      mask Display: disp('mot2_ctrl_cmd_map_Pelec_funTW_volt_in.slx')
  cstr : Subsystem
      mask Display: disp('mot2_ctrl_cstr_map_Pelec_funTW_volt_in.slx')
  dmd : Subsystem
      mask Display: disp('mot2_ctrl_dmd_uas.slx')
  system_bus_out : Outport
  local_info_bus_out : Outport  Port=2
  wires:
  [dmd] -> buscreator_system_bus_out1/3  "dmd"
  [cstr] -> buscreator_system_bus_out1/2  "cstr"
  [cmd] -> buscreator_system_bus_out1/1  "cmd"
  buscreator_system_bus_out1/1 -> system_bus_out/1
  local_info_bus_in/1 -> [local_info_bus]
  main_info_bus_in/1 -> [main_info_bus]
  [main_info_bus] -> cmd/1(inport-main_info_bus-1)
  [local_info_bus] -> cmd/2(aInport--2)
  cmd/1(outport-system_info_bus) -> [cmd], local_info_bus_out/1
  [main_info_bus] -> cstr/1(inport-main_info_bus-1)
  [local_info_bus] -> cstr/2(aInport--2)
  cstr/2(outport-cstr_bus) -> cmd/3(aInport--3)
  cstr/1(outport-system_info_bus) -> [cstr]
  [main_info_bus] -> dmd/1(inport-main_info_bus-1)
  [local_info_bus] -> dmd/2(aInport--2)
  dmd/2(outport-dmd_bus) -> cstr/3(aInport--3), cmd/4(aInport--4)
  dmd/1(outport-system_info_bus) -> [dmd]

== system AeroPropRefFranc/Propulsion and Aerodynamic Forces and Moments/S-Function/Battery Model/powerplant/mot2/plant ==
  aInport--1 : Inport
  inport-ctrl_bus-2 : Inport  Port=2
  in-effort-2 : Inport  Port=3
  in-flow-3 : Inport  Port=4
  Ground_1 : Ground
  Terminator_1 : Terminator
  mot2_plant_map_Pelec_funTW_volt_in : Subsystem
  parameter_out : Subsystem
  parameter_selection : Subsystem
  outport-system_info_bus : Outport
  outport-plant_bus : Outport  Port=2
  out-effort-7 : Outport  Port=3
  out-flow-8 : Outport  Port=4
  wires:
  Ground_1/1 -> parameter_selection/1(Inport_1)
  aInport--1/1 -> Terminator_1/1
  mot2_plant_map_Pelec_funTW_volt_in/8(mot_current_out) -> out-flow-8/1
  mot2_plant_map_Pelec_funTW_volt_in/7(mot_trq_out mot_inertia_out) -> out-effort-7/1
  in-flow-3/1 -> mot2_plant_map_Pelec_funTW_volt_in/3(spd)
  in-effort-2/1 -> mot2_plant_map_Pelec_funTW_volt_in/2(voltage)
  parameter_selection/1(outport-mot2_ctrl_cmd_simu-1) -> mot2_plant_map_Pelec_funTW_volt_in/1(mot_ctrl_cmd_simu)
  mot2_plant_map_Pelec_funTW_volt_in/6(mot_plant_temp_coeff_simu) -> parameter_out/6(inport-mot2_plant_temp_coeff_simu)
  mot2_plant_map_Pelec_funTW_volt_in/5(mot_plant_trq_out_simu) -> parameter_out/5(inport-mot2_plant_trq_out_simu)
  mot2_plant_map_Pelec_funTW_volt_in/4(mot_plant_cmd_simu) -> parameter_out/4(inport-mot2_plant_cmd_simu)
  mot2_plant_map_Pelec_funTW_volt_in/3(mot_plant_volt_in_simu) -> parameter_out/3(inport-mot2_plant_volt_in_simu)
  mot2_plant_map_Pelec_funTW_volt_in/2(mot_plant_curr_in_simu) -> parameter_out/2(inport-mot2_plant_curr_in_simu)
  mot2_plant_map_Pelec_funTW_volt_in/1(mot_plant_spd_out_simu) -> parameter_out/1(inport-mot2_plant_spd_out_simu)
  parameter_out/2(outport-plant_bus) -> outport-plant_bus/1
  parameter_out/1(outport-system_info_bus) -> outport-system_info_bus/1
  inport-ctrl_bus-2/1 -> parameter_selection/2(inport-ctrl_bus-2)

== system AeroPropRefFranc/Propulsion and Aerodynamic Forces and Moments/S-Function/Battery Model/powerplant/mot3/ctrl ==
  main_info_bus_in : Inport
  local_info_bus_in : Inport  Port=2
  buscreator_system_bus_out1 : BusCreator  Inputs=3
  cmd : Subsystem
      mask Display: disp('mot3_ctrl_cmd_map_Pelec_funTW_volt_in.slx')
  cstr : Subsystem
      mask Display: disp('mot3_ctrl_cstr_map_Pelec_funTW_volt_in.slx')
  dmd : Subsystem
      mask Display: disp('mot3_ctrl_dmd_uas.slx')
  system_bus_out : Outport
  local_info_bus_out : Outport  Port=2
  wires:
  [dmd] -> buscreator_system_bus_out1/3  "dmd"
  [cstr] -> buscreator_system_bus_out1/2  "cstr"
  [cmd] -> buscreator_system_bus_out1/1  "cmd"
  buscreator_system_bus_out1/1 -> system_bus_out/1
  local_info_bus_in/1 -> [local_info_bus]
  main_info_bus_in/1 -> [main_info_bus]
  [main_info_bus] -> cmd/1(inport-main_info_bus-1)
  [local_info_bus] -> cmd/2(aInport--2)
  cmd/1(outport-system_info_bus) -> [cmd], local_info_bus_out/1
  [main_info_bus] -> cstr/1(inport-main_info_bus-1)
  [local_info_bus] -> cstr/2(aInport--2)
  cstr/2(outport-cstr_bus) -> cmd/3(aInport--3)
  cstr/1(outport-system_info_bus) -> [cstr]
  [main_info_bus] -> dmd/1(inport-main_info_bus-1)
  [local_info_bus] -> dmd/2(aInport--2)
  dmd/2(outport-dmd_bus) -> cstr/3(aInport--3), cmd/4(aInport--4)
  dmd/1(outport-system_info_bus) -> [dmd]

== system AeroPropRefFranc/Propulsion and Aerodynamic Forces and Moments/S-Function/Battery Model/powerplant/mot3/plant ==
  aInport--1 : Inport
  inport-ctrl_bus-2 : Inport  Port=2
  in-effort-2 : Inport  Port=3
  in-flow-3 : Inport  Port=4
  Ground_1 : Ground
  Terminator_1 : Terminator
  mot3_plant_map_Pelec_funTW_volt_in : Subsystem
  parameter_out : Subsystem
  parameter_selection : Subsystem
  outport-system_info_bus : Outport
  outport-plant_bus : Outport  Port=2
  out-effort-7 : Outport  Port=3
  out-flow-8 : Outport  Port=4
  wires:
  Ground_1/1 -> parameter_selection/1(Inport_1)
  aInport--1/1 -> Terminator_1/1
  mot3_plant_map_Pelec_funTW_volt_in/8(mot_current_out) -> out-flow-8/1
  mot3_plant_map_Pelec_funTW_volt_in/7(mot_trq_out mot_inertia_out) -> out-effort-7/1
  in-flow-3/1 -> mot3_plant_map_Pelec_funTW_volt_in/3(spd)
  in-effort-2/1 -> mot3_plant_map_Pelec_funTW_volt_in/2(voltage)
  parameter_selection/1(outport-mot3_ctrl_cmd_simu-1) -> mot3_plant_map_Pelec_funTW_volt_in/1(mot_ctrl_cmd_simu)
  mot3_plant_map_Pelec_funTW_volt_in/6(mot_plant_temp_coeff_simu) -> parameter_out/6(inport-mot3_plant_temp_coeff_simu)
  mot3_plant_map_Pelec_funTW_volt_in/5(mot_plant_trq_out_simu) -> parameter_out/5(inport-mot3_plant_trq_out_simu)
  mot3_plant_map_Pelec_funTW_volt_in/4(mot_plant_cmd_simu) -> parameter_out/4(inport-mot3_plant_cmd_simu)
  mot3_plant_map_Pelec_funTW_volt_in/3(mot_plant_volt_in_simu) -> parameter_out/3(inport-mot3_plant_volt_in_simu)
  mot3_plant_map_Pelec_funTW_volt_in/2(mot_plant_curr_in_simu) -> parameter_out/2(inport-mot3_plant_curr_in_simu)
  mot3_plant_map_Pelec_funTW_volt_in/1(mot_plant_spd_out_simu) -> parameter_out/1(inport-mot3_plant_spd_out_simu)
  parameter_out/2(outport-plant_bus) -> outport-plant_bus/1
  parameter_out/1(outport-system_info_bus) -> outport-system_info_bus/1
  inport-ctrl_bus-2/1 -> parameter_selection/2(inport-ctrl_bus-2)

== system AeroPropRefFranc/Propulsion and Aerodynamic Forces and Moments/S-Function/Battery Model/powerplant/mot4/ctrl ==
  main_info_bus_in : Inport
  local_info_bus_in : Inport  Port=2
  buscreator_system_bus_out1 : BusCreator  Inputs=3
  cmd : Subsystem
      mask Display: disp('mot4_ctrl_cmd_map_Pelec_funTW_volt_in.slx')
  cstr : Subsystem
      mask Display: disp('mot4_ctrl_cstr_map_Pelec_funTW_volt_in.slx')
  dmd : Subsystem
      mask Display: disp('mot4_ctrl_dmd_uas.slx')
  system_bus_out : Outport
  local_info_bus_out : Outport  Port=2
  wires:
  [dmd] -> buscreator_system_bus_out1/3  "dmd"
  [cstr] -> buscreator_system_bus_out1/2  "cstr"
  [cmd] -> buscreator_system_bus_out1/1  "cmd"
  buscreator_system_bus_out1/1 -> system_bus_out/1
  local_info_bus_in/1 -> [local_info_bus]
  main_info_bus_in/1 -> [main_info_bus]
  [main_info_bus] -> cmd/1(inport-main_info_bus-1)
  [local_info_bus] -> cmd/2(aInport--2)
  cmd/1(outport-system_info_bus) -> [cmd], local_info_bus_out/1
  [main_info_bus] -> cstr/1(inport-main_info_bus-1)
  [local_info_bus] -> cstr/2(aInport--2)
  cstr/2(outport-cstr_bus) -> cmd/3(aInport--3)
  cstr/1(outport-system_info_bus) -> [cstr]
  [main_info_bus] -> dmd/1(inport-main_info_bus-1)
  [local_info_bus] -> dmd/2(aInport--2)
  dmd/2(outport-dmd_bus) -> cstr/3(aInport--3), cmd/4(aInport--4)
  dmd/1(outport-system_info_bus) -> [dmd]
